simulink model "NLGuidance_12B"  (Simulink 8.0)
settings: Solver=ode3  StartTime=0.0  StopTime=10.0  FixedStep=.02  RelTol=1e-3
settings Model: Creator=elliocm  LastModifiedBy=elliocm
settings DataIOCC: SignalLoggingSaveFormat=ModelDataLogs
settings DebuggingCC: MultiTaskDSMMsg=warning  MultiTaskCondExecSysMsg=none  StrictBusMsg=None
settings RTWCC: IncludeERTFirstTime=on
settings CodeAppCC: CustomSymbolStrType=$N$R$M_T  InternalIdentifier=Shortened
settings GRTTargetCC: CodeReplacementLibrary=None  CPPClassGenCompliant=on

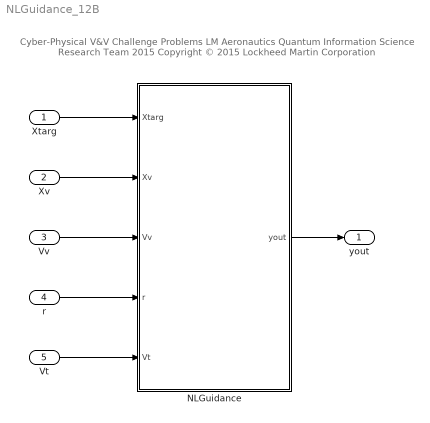
== system NLGuidance_12B ==
  note: Cyber-Physical V&V Challenge Problems
      | LM Aeronautics Quantum Information Science Research Team 2015
      | Copyright © 2015 Lockheed Martin Corporation
  Xtarg : Inport  OutDataTypeStr=double  PortDimensions=3
  Xv : Inport  Port=2  OutDataTypeStr=double  PortDimensions=3
  Vv : Inport  Port=3  OutDataTypeStr=double  PortDimensions=3
  r : Inport  Port=4  OutDataTypeStr=double
  Vt : Inport  Port=5  OutDataTypeStr=double  PortDimensions=3
  NLGuidance : Subsystem
  yout : Outport
  wires:
  NLGuidance/1(yout) -> yout/1
  Xtarg/1 -> NLGuidance/1(Xtarg)
  Xv/1 -> NLGuidance/2(Xv)
  Vv/1 -> NLGuidance/3(Vv)
  r/1 -> NLGuidance/4(r)
  Vt/1 -> NLGuidance/5(Vt)

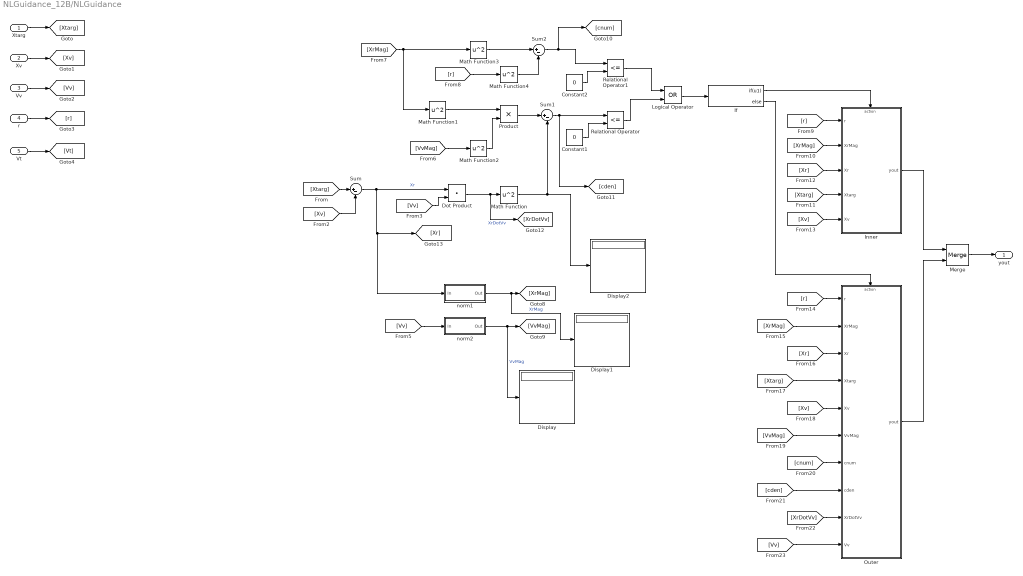
== system NLGuidance_12B/NLGuidance ==
  Xtarg : Inport
  Xv : Inport  Port=2
  Vv : Inport  Port=3
  r : Inport  Port=4
  Vt : Inport  Port=5
  Constant1 : Constant  Value=0
  Constant2 : Constant  Value=0
  Display : Display
  Display1 : Display
  Display2 : Display
  Dot Product : DotProduct  InputSameDT=on  OutDataTypeStr=Inherit: Inherit via internal rule
  If : If  IfExpression=u1
  Inner : Subsystem
  Logical Operator : Logic  Operator=OR  AllPortsSameDT=off  OutDataTypeStr=boolean
  Math Function{,1..4} (5 alike) : Math  Operator=square  SaturateOnIntegerOverflow=on
  Merge : Merge
  Outer : Subsystem
  Product : Product  RndMeth=Zero
  Relational Operator : RelationalOperator  Operator=<=  OutDataTypeStr=boolean
  Relational Operator1 : RelationalOperator  Operator=<=  OutDataTypeStr=boolean
  Sum : Sum  Inputs=|+-
  Sum1 : Sum  Inputs=|+-
  Sum2 : Sum  Inputs=|+-
  norm1 : Subsystem
  norm2 : Subsystem
  yout : Outport
  wires:
  Xtarg/1 -> [Xtarg]
  Xv/1 -> [Xv]
  Vv/1 -> [Vv]
  r/1 -> [r]
  Vt/1 -> [Vt]
  [Xtarg] -> Sum/1
  [Xv] -> Sum/2
  Sum/1 -> norm1/1(In), [Xr], Dot Product/1  "Xr"
  [Vv] -> Dot Product/2
  Dot Product/1 -> [XrDotVv], Math Function/1  "XrDotVv"
  norm1/1(Out) -> Display1/1, [XrMag]  "XrMag"
  [Vv] -> norm2/1(In)
  norm2/1(Out) -> Display/1, [VvMag]  "VvMag"
  Math Function/1 -> Display2/1, Sum1/2
  [VvMag] -> Math Function2/1
  Math Function1/1 -> Product/1
  Math Function2/1 -> Product/2
  Product/1 -> Sum1/1
  Sum1/1 -> [cden], Relational Operator/1
  Constant1/1 -> Relational Operator/2
  Relational Operator/1 -> Logical Operator/2
  Sum2/1 -> [cnum], Relational Operator1/1
  Constant2/1 -> Relational Operator1/2
  Relational Operator1/1 -> Logical Operator/1
  Math Function3/1 -> Sum2/1
  [XrMag] -> Math Function1/1, Math Function3/1
  Math Function4/1 -> Sum2/2
  [r] -> Math Function4/1
  [r] -> Inner/1(r)
  [XrMag] -> Inner/2(XrMag)
  Logical Operator/1 -> If/1
  [Xtarg] -> Inner/4(Xtarg)
  [Xr] -> Inner/3(Xr)
  [Xv] -> Inner/5(Xv)
  Inner/1(yout) -> Merge/1
  Outer/1(yout) -> Merge/2
  If/1 -> Inner/Action
  If/2 -> Outer/Action
  [r] -> Outer/1(r)
  [XrMag] -> Outer/2(XrMag)
  [Xr] -> Outer/3(Xr)
  [Xtarg] -> Outer/4(Xtarg)
  [Xv] -> Outer/5(Xv)
  [VvMag] -> Outer/6(VvMag)
  [cnum] -> Outer/7(cnum)
  [cden] -> Outer/8(cden)
  [XrDotVv] -> Outer/9(XrDotVv)
  [Vv] -> Outer/10(Vv)
  Merge/1 -> yout/1

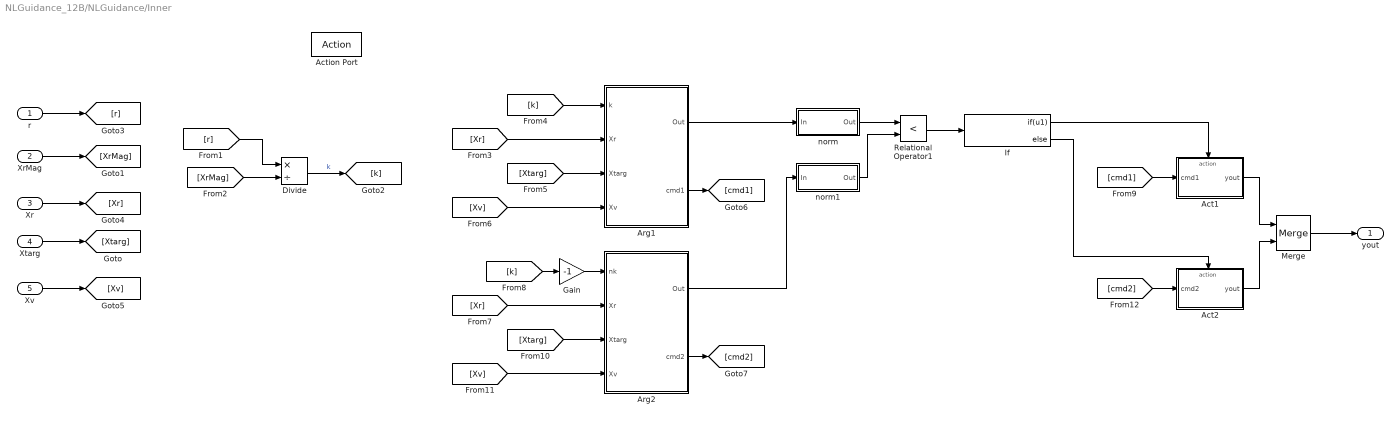
== system NLGuidance_12B/NLGuidance/Inner ==
  r : Inport
  XrMag : Inport  Port=2
  Xr : Inport  Port=3
  Xtarg : Inport  Port=4
  Xv : Inport  Port=5
  Action Port : ActionPort  ActionType=then
  Act1 : Subsystem
  Act2 : Subsystem
  Arg1 : Subsystem
  Arg2 : Subsystem
  Divide : Product  Inputs=*/
  Gain : Gain  Gain=-1
  If : If  IfExpression=u1
  Merge : Merge
  Relational Operator1 : RelationalOperator  Operator=<  OutDataTypeStr=boolean
  norm : Subsystem
  norm1 : Subsystem
  yout : Outport
  wires:
  Divide/1 -> [k]  "k"
  r/1 -> [r]
  XrMag/1 -> [XrMag]
  Xtarg/1 -> [Xtarg]
  [r] -> Divide/1
  [XrMag] -> Divide/2
  Xr/1 -> [Xr]
  Xv/1 -> [Xv]
  norm/1(Out) -> Relational Operator1/1
  norm1/1(Out) -> Relational Operator1/2
  Arg1/1(Out) -> norm/1(In)
  [k] -> Arg1/1(k)
  [Xr] -> Arg1/2(Xr)
  [Xtarg] -> Arg1/3(Xtarg)
  [Xv] -> Arg1/4(Xv)
  Relational Operator1/1 -> If/1
  [Xr] -> Arg2/2(Xr)
  [Xtarg] -> Arg2/3(Xtarg)
  [Xv] -> Arg2/4(Xv)
  Arg2/1(Out) -> norm1/1(In)
  [k] -> Gain/1
  Gain/1 -> Arg2/1(nk)
  Arg1/2(cmd1) -> [cmd1]
  Arg2/2(cmd2) -> [cmd2]
  [cmd1] -> Act1/1(cmd1)
  [cmd2] -> Act2/1(cmd2)
  Act1/1(yout) -> Merge/1
  Act2/1(yout) -> Merge/2
  Merge/1 -> yout/1
  If/1 -> Act1/Action
  If/2 -> Act2/Action

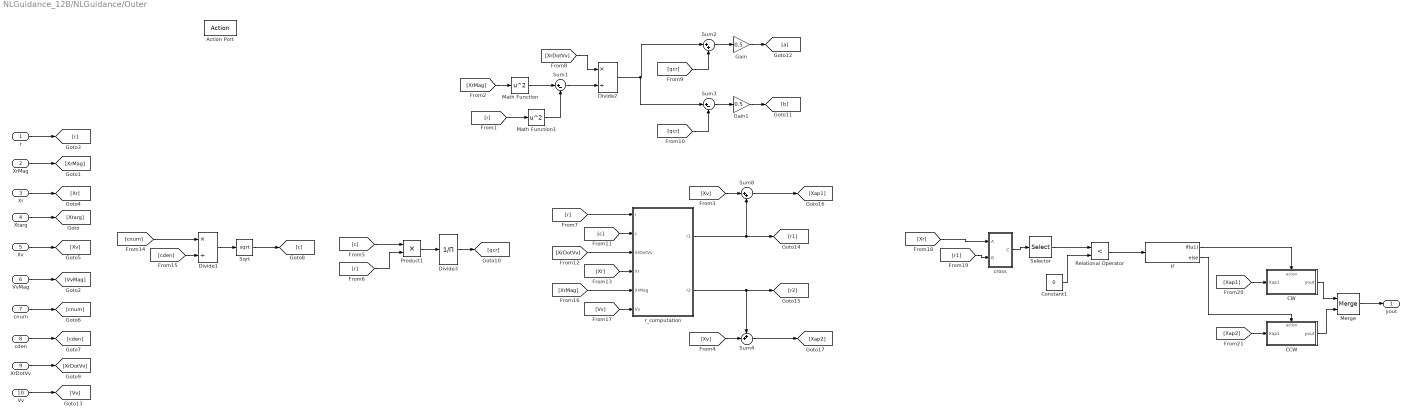
== system NLGuidance_12B/NLGuidance/Outer ==
  r : Inport
  XrMag : Inport  Port=2
  Xr : Inport  Port=3
  Xtarg : Inport  Port=4
  Xv : Inport  Port=5
  VvMag : Inport  Port=6
  cnum : Inport  Port=7
  cden : Inport  Port=8
  XrDotVv : Inport  Port=9
  Vv : Inport  Port=10
  Action Port : ActionPort  ActionType=else
  CCW : Subsystem
  CW : Subsystem
  Constant1 : Constant  Value=0
  Divide1 : Product  Inputs=*/
  Divide2 : Product  Inputs=*/
  Divide3 : Product  Inputs=/
  Gain : Gain  Gain=0.5
  Gain1 : Gain  Gain=0.5
  If : If  IfExpression=u1
  Math Function : Math  Operator=square  SaturateOnIntegerOverflow=on
  Math Function1 : Math  Operator=square  SaturateOnIntegerOverflow=on
  Merge : Merge
  Product1 : Product
  Relational Operator : RelationalOperator  Operator=<  OutDataTypeStr=boolean
  Selector : Selector  InputPortWidth=3  IndexOptions=Index vector (dialog)  Indices=[3]  OutputSizes=1
  Sqrt : Sqrt  SaturateOnIntegerOverflow=on
  Sum1 : Sum  Inputs=|+-
  Sum2 : Sum  Inputs=|++
  Sum3 : Sum  Inputs=|+-
  Sum4 : Sum  Inputs=++|
  Sum8 : Sum  Inputs=|++
  cross : Subsystem
  r_computation : Subsystem
  yout : Outport
  wires:
  r/1 -> [r]
  XrMag/1 -> [XrMag]
  Xtarg/1 -> [Xtarg]
  Xr/1 -> [Xr]
  Xv/1 -> [Xv]
  [XrMag] -> Math Function/1
  [r] -> Math Function1/1
  VvMag/1 -> [VvMag]
  cnum/1 -> [cnum]
  [cnum] -> Divide1/1
  [cden] -> Divide1/2
  Divide1/1 -> Sqrt/1
  Sqrt/1 -> [c]
  cden/1 -> [cden]
  XrDotVv/1 -> [XrDotVv]
  [c] -> Product1/1
  [r] -> Product1/2
  Math Function/1 -> Sum1/1
  Math Function1/1 -> Sum1/2
  Sum1/1 -> Divide2/2
  [XrDotVv] -> Divide2/1
  Divide2/1 -> Sum3/1, Sum2/1
  Sum2/1 -> Gain/1
  Sum3/1 -> Gain1/1
  Product1/1 -> Divide3/1
  Divide3/1 -> [qcr]
  [qcr] -> Sum2/2
  [qcr] -> Sum3/2
  Gain1/1 -> [b]
  Gain/1 -> [a]
  Vv/1 -> [Vv]
  r_computation/1(r1) -> Sum8/2, [r1]
  r_computation/2(r2) -> Sum4/1, [r2]
  [Xv] -> Sum8/1
  [Xv] -> Sum4/2
  Sum8/1 -> [Xap1]
  Sum4/1 -> [Xap2]
  [r] -> r_computation/1(r)
  [c] -> r_computation/2(c)
  [XrDotVv] -> r_computation/3(XrDotVv)
  [Xr] -> r_computation/4(Xr)
  [XrMag] -> r_computation/5(XrMag)
  [Vv] -> r_computation/6(Vv)
  cross/1(C) -> Selector/1
  [Xr] -> cross/1(A)
  [r1] -> cross/2(B)
  Constant1/1 -> Relational Operator/2
  Selector/1 -> Relational Operator/1
  Relational Operator/1 -> If/1
  If/1 -> CW/Action
  [Xap1] -> CW/1(Xap1)
  If/2 -> CCW/Action
  [Xap2] -> CCW/1(Xap1)
  CW/1(yout) -> Merge/1
  CCW/1(yout) -> Merge/2
  Merge/1 -> yout/1

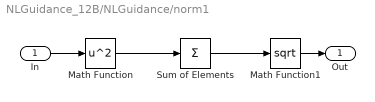
== system NLGuidance_12B/NLGuidance/norm1 ==
  In : Inport
  Math Function : Math  Operator=square  SaturateOnIntegerOverflow=on
  Math Function1 : Math  Operator=sqrt  SaturateOnIntegerOverflow=on
  Sum of Elements : Sum  Inputs=+
  Out : Outport
  wires:
  Math Function/1 -> Sum of Elements/1
  Sum of Elements/1 -> Math Function1/1
  In/1 -> Math Function/1
  Math Function1/1 -> Out/1

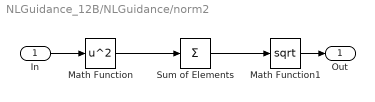
== system NLGuidance_12B/NLGuidance/norm2 ==
  In : Inport
  Math Function : Math  Operator=square  SaturateOnIntegerOverflow=on
  Math Function1 : Math  Operator=sqrt  SaturateOnIntegerOverflow=on
  Sum of Elements : Sum  Inputs=+
  Out : Outport
  wires:
  Math Function1/1 -> Out/1
  In/1 -> Math Function/1
  Sum of Elements/1 -> Math Function1/1
  Math Function/1 -> Sum of Elements/1

== system NLGuidance_12B/NLGuidance/Inner/Act1 ==
  cmd1 : Inport
  Action Port : ActionPort  ActionType=then
  yout : Outport
  wires:
  cmd1/1 -> yout/1

== system NLGuidance_12B/NLGuidance/Inner/Act2 ==
  cmd2 : Inport
  Action Port : ActionPort  ActionType=else
  yout : Outport
  wires:
  cmd2/1 -> yout/1

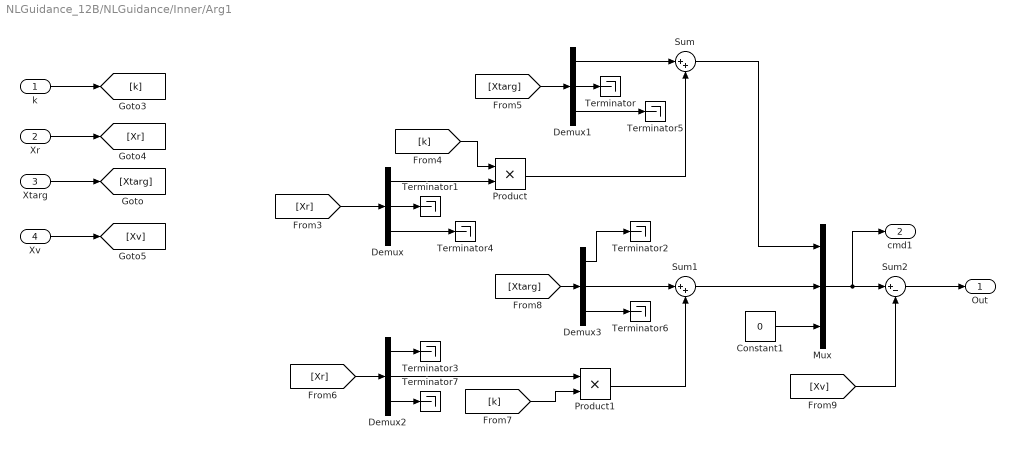
== system NLGuidance_12B/NLGuidance/Inner/Arg1 ==
  k : Inport
  Xr : Inport  Port=2
  Xtarg : Inport  Port=3
  Xv : Inport  Port=4
  Constant1 : Constant  Value=0
  Demux{,1..3} (4 alike) : Demux  Outputs=3
  Mux : Mux  Inputs=3
  Product : Product  RndMeth=Zero
  Product1 : Product  RndMeth=Zero
  Sum : Sum  Inputs=|++
  Sum1 : Sum  Inputs=|++
  Sum2 : Sum  Inputs=|+-
  Terminator{,1..7} (8 alike) : Terminator
  Out : Outport
  cmd1 : Outport  Port=2
  wires:
  Mux/1 -> cmd1/1, Sum2/1
  Demux3/3 -> Terminator6/1
  Demux/2 -> Terminator1/1
  [Xr] -> Demux2/1
  Sum/1 -> Mux/1
  Demux1/2 -> Terminator/1
  [k] -> Product1/2
  Constant1/1 -> Mux/3
  Demux3/2 -> Sum1/1
  Demux2/1 -> Terminator3/1
  [Xtarg] -> Demux1/1
  Product/1 -> Sum/2
  [k] -> Product/1
  Demux/1 -> Product/2
  [Xr] -> Demux/1
  Sum1/1 -> Mux/2
  Demux1/1 -> Sum/1
  Demux2/3 -> Terminator7/1
  [Xtarg] -> Demux3/1
  Sum2/1 -> Out/1
  Demux/3 -> Terminator4/1
  [Xv] -> Sum2/2
  Demux3/1 -> Terminator2/1
  Demux2/2 -> Product1/1
  Product1/1 -> Sum1/2
  Demux1/3 -> Terminator5/1
  k/1 -> [k]
  Xtarg/1 -> [Xtarg]
  Xr/1 -> [Xr]
  Xv/1 -> [Xv]

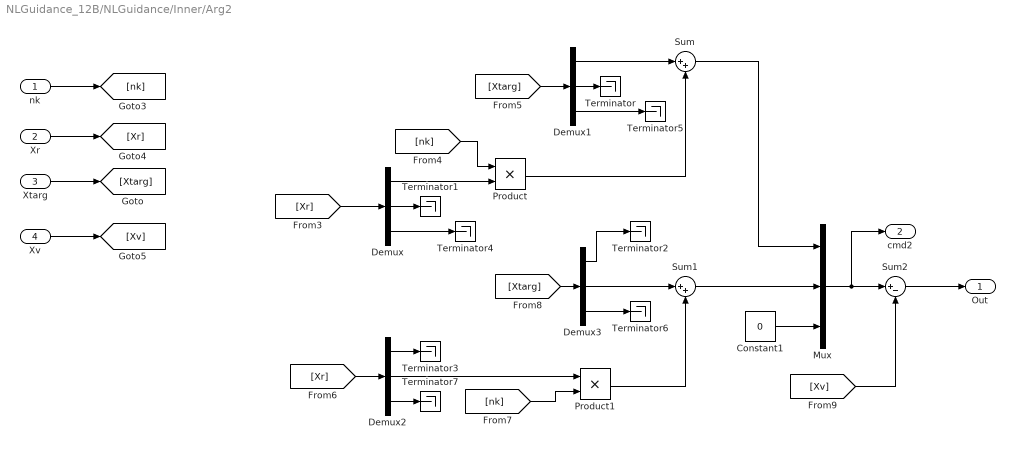
== system NLGuidance_12B/NLGuidance/Inner/Arg2 ==
  nk : Inport
  Xr : Inport  Port=2
  Xtarg : Inport  Port=3
  Xv : Inport  Port=4
  Constant1 : Constant  Value=0
  Demux{,1..3} (4 alike) : Demux  Outputs=3
  Mux : Mux  Inputs=3
  Product : Product  RndMeth=Zero
  Product1 : Product  RndMeth=Zero
  Sum : Sum  Inputs=|++
  Sum1 : Sum  Inputs=|++
  Sum2 : Sum  Inputs=|+-
  Terminator{,1..7} (8 alike) : Terminator
  Out : Outport
  cmd2 : Outport  Port=2
  wires:
  Xv/1 -> [Xv]
  Xr/1 -> [Xr]
  Xtarg/1 -> [Xtarg]
  nk/1 -> [nk]
  Demux1/3 -> Terminator5/1
  Product1/1 -> Sum1/2
  Demux2/2 -> Product1/1
  Demux3/1 -> Terminator2/1
  [Xv] -> Sum2/2
  Demux/3 -> Terminator4/1
  Sum2/1 -> Out/1
  [Xtarg] -> Demux3/1
  Demux2/3 -> Terminator7/1
  Demux1/1 -> Sum/1
  Sum1/1 -> Mux/2
  [Xr] -> Demux/1
  Demux/1 -> Product/2
  [nk] -> Product/1
  Product/1 -> Sum/2
  [Xtarg] -> Demux1/1
  Demux2/1 -> Terminator3/1
  Demux3/2 -> Sum1/1
  Constant1/1 -> Mux/3
  [nk] -> Product1/2
  Demux1/2 -> Terminator/1
  Sum/1 -> Mux/1
  [Xr] -> Demux2/1
  Demux/2 -> Terminator1/1
  Demux3/3 -> Terminator6/1
  Mux/1 -> cmd2/1, Sum2/1

== system NLGuidance_12B/NLGuidance/Inner/norm ==
  In : Inport
  Math Function : Math  Operator=square  SaturateOnIntegerOverflow=on
  Math Function1 : Math  Operator=sqrt  SaturateOnIntegerOverflow=on
  Sum of Elements : Sum  Inputs=+
  Out : Outport
  wires:
  Math Function1/1 -> Out/1
  In/1 -> Math Function/1
  Sum of Elements/1 -> Math Function1/1
  Math Function/1 -> Sum of Elements/1

== system NLGuidance_12B/NLGuidance/Inner/norm1 ==
  In : Inport
  Math Function : Math  Operator=square  SaturateOnIntegerOverflow=on
  Math Function1 : Math  Operator=sqrt  SaturateOnIntegerOverflow=on
  Sum of Elements : Sum  Inputs=+
  Out : Outport
  wires:
  Math Function/1 -> Sum of Elements/1
  Sum of Elements/1 -> Math Function1/1
  In/1 -> Math Function/1
  Math Function1/1 -> Out/1

== system NLGuidance_12B/NLGuidance/Outer/CCW ==
  Xap1 : Inport
  Action Port : ActionPort  ActionType=else
  yout : Outport
  wires:
  Xap1/1 -> yout/1

== system NLGuidance_12B/NLGuidance/Outer/CW ==
  Xap1 : Inport
  Action Port : ActionPort  ActionType=then
  yout : Outport
  wires:
  Xap1/1 -> yout/1

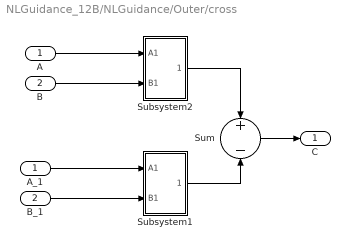
== system NLGuidance_12B/NLGuidance/Outer/cross ==
  A : Inport
  B : Inport  Port=2
  A_1 : InportShadow
  B_1 : InportShadow  Port=2
  Subsystem1 : Subsystem
  Subsystem2 : Subsystem
  Sum : Sum  Inputs=+|-  SaturateOnIntegerOverflow=on  InputSameDT=on  OutDataTypeStr=Inherit: Same as first input
  C : Outport
  wires:
  B/1 -> Subsystem2/2(B1)
  A_1/1 -> Subsystem1/1(A1)
  A/1 -> Subsystem2/1(A1)
  Subsystem2/1(Out1) -> Sum/1
  B_1/1 -> Subsystem1/2(B1)
  Sum/1 -> C/1
  Subsystem1/1(Out1) -> Sum/2

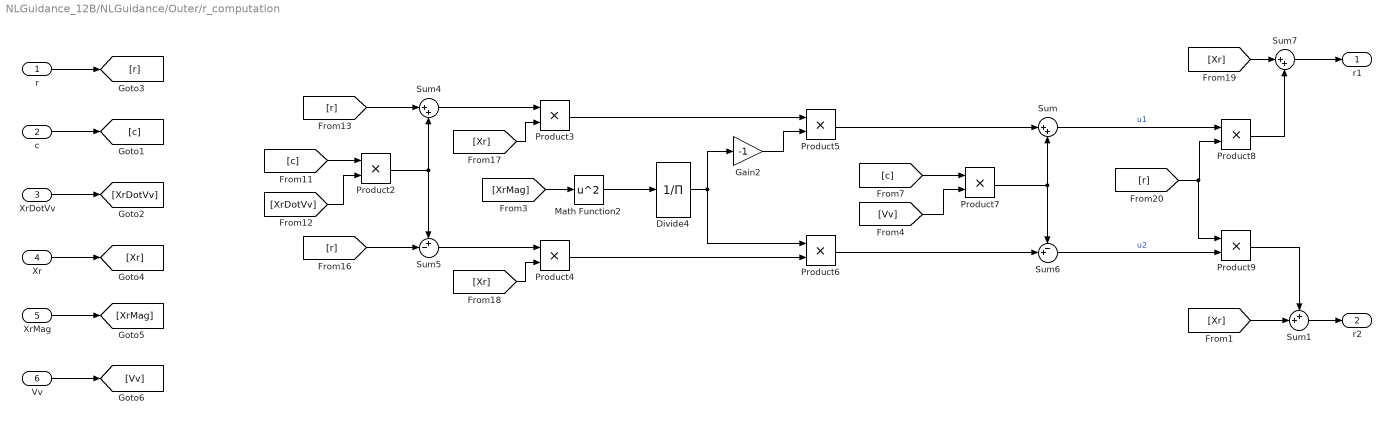
== system NLGuidance_12B/NLGuidance/Outer/r_computation ==
  r : Inport
  c : Inport  Port=2
  XrDotVv : Inport  Port=3
  Xr : Inport  Port=4
  XrMag : Inport  Port=5
  Vv : Inport  Port=6
  Divide4 : Product  Inputs=/
  Gain2 : Gain  Gain=-1
  Math Function2 : Math  Operator=square  SaturateOnIntegerOverflow=on
  Product{2..9} (8 alike) : Product
  Sum : Sum  Inputs=|++
  Sum1 : Sum  Inputs=++|
  Sum4 : Sum  Inputs=|++
  Sum5 : Sum  Inputs=+-|
  Sum6 : Sum  Inputs=-+|
  Sum7 : Sum  Inputs=|++
  r1 : Outport
  r2 : Outport  Port=2
  wires:
  [r] -> Sum4/1
  Sum6/1 -> Product9/2  "u2"
  Gain2/1 -> Product5/2
  Product4/1 -> Product6/2
  [XrDotVv] -> Product2/2
  [Xr] -> Product4/2
  Product3/1 -> Product5/1
  Divide4/1 -> Product6/1, Gain2/1
  Sum5/1 -> Product4/1
  [Xr] -> Sum7/1
  [Vv] -> Product7/2
  Product7/1 -> Sum/2, Sum6/1
  [r] -> Product9/1, Product8/2
  Product8/1 -> Sum7/2
  Sum7/1 -> r1/1
  Product6/1 -> Sum6/2
  Product5/1 -> Sum/1
  [Xr] -> Product3/2
  [c] -> Product7/1
  Math Function2/1 -> Divide4/1
  [XrMag] -> Math Function2/1
  [c] -> Product2/1
  Sum4/1 -> Product3/1
  Sum/1 -> Product8/1  "u1"
  Product2/1 -> Sum5/1, Sum4/2
  [r] -> Sum5/2
  r/1 -> [r]
  c/1 -> [c]
  XrDotVv/1 -> [XrDotVv]
  Xr/1 -> [Xr]
  XrMag/1 -> [XrMag]
  Vv/1 -> [Vv]
  Product9/1 -> Sum1/1
  [Xr] -> Sum1/2
  Sum1/1 -> r2/1

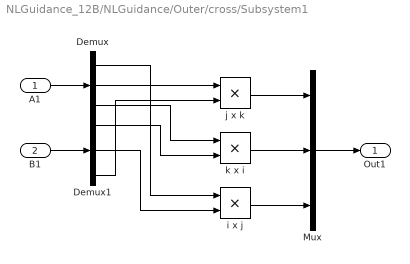
== system NLGuidance_12B/NLGuidance/Outer/cross/Subsystem1 ==
  A1 : Inport
  B1 : Inport  Port=2
  Demux : Demux  Outputs=3
  Demux1 : Demux  Outputs=3
  Mux : Mux  Inputs=3
  i x j : Product  SaturateOnIntegerOverflow=on  InputSameDT=on  OutDataTypeStr=Inherit: Same as first input
  j x k : Product  SaturateOnIntegerOverflow=on  InputSameDT=on  OutDataTypeStr=Inherit: Same as first input
  k x i : Product  SaturateOnIntegerOverflow=on  InputSameDT=on  OutDataTypeStr=Inherit: Same as first input
  Out1 : Outport
  wires:
  Demux/2 -> j x k/1
  Demux1/3 -> j x k/2
  A1/1 -> Demux/1
  Demux/3 -> k x i/1
  Mux/1 -> Out1/1
  j x k/1 -> Mux/1
  B1/1 -> Demux1/1
  k x i/1 -> Mux/2
  Demux1/2 -> i x j/2
  i x j/1 -> Mux/3
  Demux/1 -> i x j/1
  Demux1/1 -> k x i/2

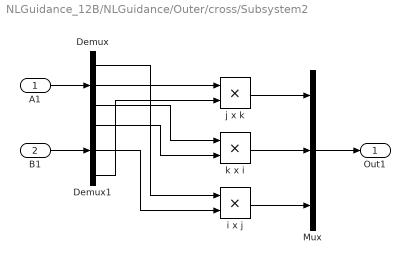
== system NLGuidance_12B/NLGuidance/Outer/cross/Subsystem2 ==
  A1 : Inport
  B1 : Inport  Port=2
  Demux : Demux  Outputs=3
  Demux1 : Demux  Outputs=3
  Mux : Mux  Inputs=3
  i x j : Product  SaturateOnIntegerOverflow=on  InputSameDT=on  OutDataTypeStr=Inherit: Same as first input
  j x k : Product  SaturateOnIntegerOverflow=on  InputSameDT=on  OutDataTypeStr=Inherit: Same as first input
  k x i : Product  SaturateOnIntegerOverflow=on  InputSameDT=on  OutDataTypeStr=Inherit: Same as first input
  Out1 : Outport
  wires:
  Demux1/1 -> k x i/2
  Demux/1 -> i x j/1
  i x j/1 -> Mux/3
  Demux1/2 -> i x j/2
  k x i/1 -> Mux/2
  B1/1 -> Demux1/1
  j x k/1 -> Mux/1
  Mux/1 -> Out1/1
  Demux/3 -> k x i/1
  A1/1 -> Demux/1
  Demux1/3 -> j x k/2
  Demux/2 -> j x k/1
